simulink model "s_waag11"  (Simulink 4.00)
settings: Solver=ode15s  SolverMode=SingleTasking  StartTime=0.0  StopTime=0.5  FixedStep=1e-4  MaxStep=1e-3  RelTol=1e-3  AbsTol=1e-6
values from neighbouring files (symbols this model uses):
  D = my_sys1.d    [ncd_estim1.m]    (also in ncd_estim_1.mat = 0; ncd_kalm1.m; ncd_kalm2.m; ncd_kalm_1.mat = 0)
  g = 9.8    [ident21.mat]    (also in torce11.m = 9.81; torcell.mat = 9.81; waag11.m = 9.81; waag11.mat = 9.81)
  kg = 5    [waag11.m]    (also in waag11.mat; waage2.m; waage3.m)
  ks = 200    [waag11.m]    (also in waag11.mat; waage2.m; waage3.m = 300)
  L = place(A, B, p)'    [ncd_estim1.m]    (also in ncd_estim_1.mat = [29.04 93.6748 304.13176 464.47352 317.56952 149.5392]; ncd_kalm_2.mat = [29.04 93.6748 304.13176 464.47352 317.56952 149.5392]; torce11.m = axis; torcell.mat = [0 100 0 3])
  mw = 0.1    [waag11.m]    (also in waag11.mat; waage2.m; waage3.m = 0.5)
  mx = 5    [waag11.m]    (also in waag11.mat; waage2.m; waage3.m)
  R = 1    [ncd_estim1.m]    (also in ncd_estim_1.mat; ncd_kalm1.m; ncd_kalm2.m; ncd_kalm_1.mat)
  r = 0.0003    [ident21.mat]    (also in waag11.m = 100; waag11.mat = 100; waage2.m = 100; waage3.m = 100)
settings Model: LastModifiedBy=Administrator  SaveTime=off  SaveOutput=off  LimitDataPoints=off  BlockReductionOpt=off

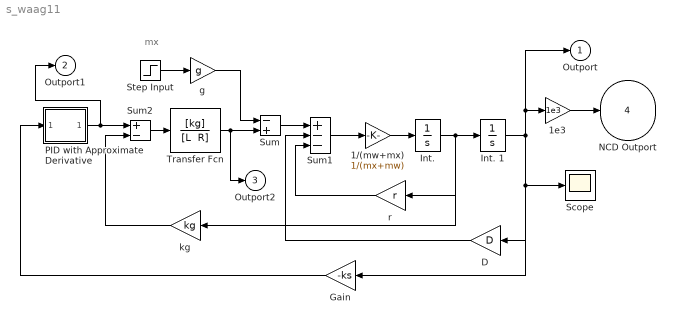
== system s_waag11 ==
  note: mx
  1/(mw+mx) : Gain  Gain=1/(mx+mw)  Multiplication=Element-wise(K.*u)  SaturateOnIntegerOverflow=on
  1e3 : Gain  Gain=1e3  Multiplication=Element-wise(K.*u)  SaturateOnIntegerOverflow=on
  D : Gain  Orientation=left  Gain=D  Multiplication=Element-wise(K.*u)  SaturateOnIntegerOverflow=on
  Gain : Gain  Orientation=left  Gain=-ks  Multiplication=Element-wise(K.*u)  SaturateOnIntegerOverflow=on
  Int. : Integrator  ExternalReset=none  InitialConditionSource=internal  InitialCondition=0  LimitOutput=off  UpperSaturationLimit=inf  LowerSaturationLimit=-inf  ShowSaturationPort=off  ShowStatePort=off  AbsoluteTolerance=auto
  Int. 1 : Integrator  ExternalReset=none  InitialConditionSource=internal  InitialCondition=0  LimitOutput=off  UpperSaturationLimit=inf  LowerSaturationLimit=-inf  ShowSaturationPort=off  ShowStatePort=off  AbsoluteTolerance=auto
  PID with Approximate Derivative : Subsystem  mask(PID(2) Controller){@1=kp, @2=ki, @3=kd, @4=N}
      mask prompts: @1 "Proportional:"; @2 "Integral"; @3 "Derivative:"; @4 "Derivative divisor(N):"
      mask help:
      | Enter Proportional(P), Integral(I), and Derivative(D) and divisor (N) terms.
      | P+I/s+Ds/(1/Ns+1)
      mask init:
      | P=@1; I=@2; D=@3; N=@4;
      settings: RTWFcnNameOpts=Auto  RTWFileNameOpts=Auto
      mask Help: This block implements a PID controller where parameters are entered for the Proportional, Integral and Derivative and divisor terms. Unmask this block to see how it works. The derivative term is implemented using an:\ns/(s/N +1)  transfer function block. Making N large can create a "stiff" system.
      mask Display: disp('PID')
  Scope : Scope
      settings: TickLabels=on  TimeRange=0.5  YMin=-0.0025  YMax=0  SaveToWorkspace=off  SaveName=ScopeData  DataFormat=Array  LimitDataPoints=on  MaxDataPoints=5000
  Step Input : Step  Time=0  Before=0  After=mx  SampleTime=0
  Sum : Sum  Inputs=-+  SaturateOnIntegerOverflow=on
  Sum1 : Sum  Inputs=+--  SaturateOnIntegerOverflow=on
  Sum2 : Sum  Inputs=+-  SaturateOnIntegerOverflow=on
  Transfer Fcn : TransferFcn  Numerator=[kg]  Denominator="[L  R]"  Realization=auto  AbsoluteTolerance=auto
  g : Gain  Gain=g  Multiplication=Element-wise(K.*u)  SaturateOnIntegerOverflow=on
  kg : Gain  Orientation=left  Gain=kg  Multiplication=Element-wise(K.*u)  SaturateOnIntegerOverflow=on
  r : Gain  Orientation=left  Gain=r  Multiplication=Element-wise(K.*u)  SaturateOnIntegerOverflow=on
  Outport : Outport  Port=1  InitialOutput=0
  Outport1 : Outport  Port=2  InitialOutput=0
  Outport2 : Outport  Port=3  InitialOutput=0
  NCD Outport : Outport  Port=4  InitialOutput=0
      settings: OpenFcn=optblock
      mask Type: NCD Outport
      mask Display:
      | plot([0:10],[-.5 1.5 .6 1.3 .8 1.1 .95 1.02 .99 1 1]);
      | disp('\n\n NCD\n OutPort 4');
  wires:
  Transfer Fcn/1 -> Outport2/1, Sum/2
  PID with Approximate Derivative/1(Out_1) -> Outport1/1, Sum2/1
  kg/1 -> Sum2/2
  Sum2/1 -> Transfer Fcn/1
  Int. 1/1 -> Scope/1, Gain/1, D/1, Outport/1, 1e3/1
  Gain/1 -> PID with Approximate Derivative/1(In_1)
  r/1 -> Sum1/3
  Int./1 -> kg/1, r/1, Int. 1/1
  D/1 -> Sum1/2
  1/(mw+mx)/1 -> Int./1
  Sum1/1 -> 1/(mw+mx)/1
  Sum/1 -> Sum1/1
  g/1 -> Sum/1
  Step Input/1 -> g/1
  1e3/1 -> NCD Outport/1

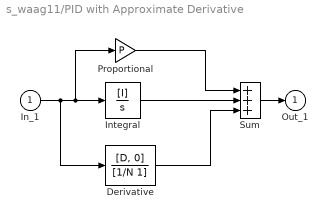
== system s_waag11/PID with Approximate Derivative ==
  In_1 : Inport  Port=1
  Derivative : TransferFcn  Numerator=[D, 0]  Denominator=[1/N 1]  Realization=auto  AbsoluteTolerance=auto
  Integral : TransferFcn  Numerator=[I]  Denominator=[1 0]  Realization=auto  AbsoluteTolerance=auto
  Proportional : Gain  Gain=P  Multiplication=Element-wise(K.*u)  SaturateOnIntegerOverflow=on
  Sum : Sum  Inputs=+++  SaturateOnIntegerOverflow=on
  Out_1 : Outport  Port=1  InitialOutput=0
  wires:
  Sum/1 -> Out_1/1
  In_1/1 -> Derivative/1, Proportional/1, Integral/1
  Derivative/1 -> Sum/3
  Integral/1 -> Sum/2
  Proportional/1 -> Sum/1
